simulink model "mpptwithANN"  (R2024b)
settings: Solver=VariableStepAuto  StartTime=0.0  StopTime=24.0  RelTol=1e-3
undefined symbols (not defined in the file): C_boost, f, L_boost, Lf, numericIrradiance, numericTemperature, PV_power_max, Ts, V_bus_ref
libraries: neural x84, slpidlib x3, spsSeriesRLCBranchLib x3, spsDiodeLib x1, spsIGBTLib x1, spsPLL3phLib x1, spsPWMGenerator2LevelLib x1, spsPower3phInstantaneousLib x1, spsTHDLib x1, spsabctodq0Lib x1, spsdq0toabcLib x1, spsThreePhaseSeriesRLCBranchLib x1
(part 3 of 3)

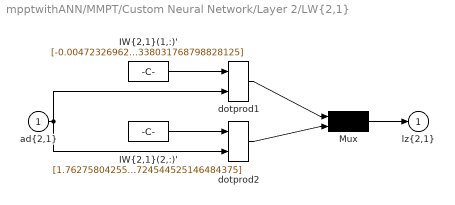
== system mpptwithANN/MMPT/Custom Neural Network/Layer 2/LW{2,1} ==
  "ad{2,1}" : Inport  PortDimensions=80
      mask Display: e = 0.06;c1 = [120 230 180]/255;c2 = ([120 230 180]+0)/(256+128);c3 = ([120 230 180]+128)/(256+128);patch([0 1 1 0],[0 0 1 1],c1);patch([0 1 1 1-e 1-e 0+e],[0 0 1 1-e 0+e 0+e],c2);patch([0 0 1 1-e 0+e 0+e],[0 1 1 1-e 1-e 0+e],c3);plot([0 1 1 0 0],[0 0 1 1 0]);
  "IW{2,1}(1,:)'" : Constant  Value=[-0.0047232696251935414599731899443213478662073612213134765625;-0.214237498205491594394089815978077240288257598876953125;-0.1861746145919385975187054782509221695363521575927734375;1.28709666919888210401268224813975393772125244140625;0.078470024721729980665685388885322026908397674560546875;1.731270590613536608515232728677801787853240966796875;1.00782466533039904987845147843472659587860107421875;1.6899709230974770957089958756114356219768524169921875;0.2274277742496670084992871352369547821581363677978515625;1.2774883926330662387016445791232399642467498779296875;1.2389200467032444041848293636576272547245025634765625;-0.6597367870607697692975079917232505977153778076171875;-0.06730057110412183962733223552277195267379283905029296875;0.24775995851258281188478349577053450047969818115234375;-1.264628121434770324782448369660414755344390869140625;0.11569644421095424957623976069953641854226589202880859375;-1.8753584133780234477484327726415358483791351318359375;0.71299671585435409060238498568651266396045684814453125;-0.6809653627305765066779486005543731153011322021484375;0.2444300914592904827582486859682830981910228729248046875;0.0794709997339119456061240498456754721701145172119140625;0.36944574372709626519650782938697375357151031494140625;0.88816890041603169247963478483143262565135955810546875;-0.02143380132873128063319967395727871917188167572021484375;0.50087358020141803383040723929298110306262969970703125;0.58260337805890072271353119504055939614772796630859375;-0.038040339388145251453554607223850325681269168853759765625;0.02344252262479391835103825769692775793373584747314453125;2.82094834954563111750758253037929534912109375;-0.04656330082969177552865147617922048084437847137451171875;1.098162614279721172039216980920173227787017822265625;0.462487932987993344280397423062822781503200531005859375;0.1327519260842389969834442808860330842435359954833984375;1.526963466155728088580190160428173840045928955078125;0.1184090589325994258285135174446622841060161590576171875;1.09930493106891535859404029906727373600006103515625;0.459243461526841978415092171417200006544589996337890625;0.040550115986065816964245556164314621128141880035400390625;0.0074893255565064709156075650753336958587169647216796875;-1.610216391686119852266756424796767532825469970703125;-0.260922289002195995077926227168063633143901824951171875;1.8914037685748421591114265538635663688182830810546875;0.029054511814582906215065349897486157715320587158203125;-1.291752843773599668253382333205081522464752197265625;-0.81151039446108785835320986734586767852306365966796875;-0.54747929068007616937308057458722032606601715087890625;0.6616069406555309395656649940065108239650726318359375;0.12428578364523527877150144149709376506507396697998046875;-0.0513260459514583156082068171599530614912509918212890625;0.26420608372235643290792950210743583738803863525390625;0.20916434229732139282731395724113099277019500732421875;-0.0612569342180534215369647199622704647481441497802734375;-1.011025237375536622863592128851450979709625244140625;0.2016605023533524221335255788289941847324371337890625;-0.070160014212906574027073247634689323604106903076171875;0.1338316497629020440651714807245298288762569427490234375;-0.1716200194942450185653370908767101354897022247314453125;-0.0084522613780383219761471735864688525907695293426513671875;-0.33277668814661753859951431877561844885349273681640625;0.40271319195953381164798656755010597407817840576171875;-1.693222936690923052793777969782240688800811767578125;2.97023091289202323395102212089113891124725341796875;0.60863251712745924937308927837875671684741973876953125;0.215351659861896804759595625000656582415103912353515625;0.199347225804359318157565894580329768359661102294921875;0.00390281946643264605889545038053256575949490070343017578125;0.155476210424553784594792205098201520740985870361328125;0.15170365314607192619433817526441998779773712158203125;0.07248701893488292136158435141624067910015583038330078125;1.544695222341591733794530227896757423877716064453125 ...(+582 chars)]
      mask Display: e = 0.06;c1 = [120 150 230]/255;c2 = ([120 150 230]+0)/383;c3 = ([120 150 230]+128)/383;patch([0 1 1 0],[0 0 1 1],c1);patch([0 1 1 1-e 1-e 0+e],[0 0 1 1-e 0+e 0+e],c2);patch([0 0 1 1-e 0+e 0+e],[0 1 1 1-e 1-e 0+e],c3);plot([0 1 1 0 0],[0 0 1 1 0]);disp('weights');
  "IW{2,1}(2,:)'" : Constant  Value=[1.7627580425513749151633646761183626949787139892578125;0.53943205208589140031705255751148797571659088134765625;0.624002903812199694044693387695588171482086181640625;-0.243051189123102251432584353096899576485157012939453125;1.1020632737466886652555331238545477390289306640625;-1.11695945169389698747863803873769938945770263671875;-0.98308582001807309769247922304202802479267120361328125;-0.057565707001347922455725125701064825989305973052978515625;1.0363818644077980035689279247890226542949676513671875;0.384261316616549664093582805435289628803730010986328125;0.3909105472417533366780162396025843918323516845703125;-1.7467929934915356060542990235262550413608551025390625;0.56609445637508437609852762761875055730342864990234375;0.265017689055616234572454459339496679604053497314453125;1.2954045387665560351564408847480081021785736083984375;-1.540932836613462253438910920522175729274749755859375;1.841363864427123520073337203939445316791534423828125;-0.305536607589804276585709885694086551666259765625;-1.13861542101164392448708895244635641574859619140625;1.625627574860612600815557016176171600818634033203125;2.8671914143540409014576653135009109973907470703125;0.346381542809648890202112170300097204744815826416015625;1.1745140811006609116162735517718829214572906494140625;-5.6920796134959150691656759590841829776763916015625;0.3262136683259966307701915866346098482608795166015625;-0.650348270424956353963352739810943603515625;3.41910464775504596701694026705808937549591064453125;-0.44059910956027170669813131098635494709014892578125;0.09728772033335808533394128971849568188190460205078125;2.2946392991425330620813838322646915912628173828125;-0.1401781681152533820533534481000970117747783660888671875;-6.91661892860060145693523736554197967052459716796875;1.0106115736624785572672635680646635591983795166015625;0.403771461315584889728569351063924841582775115966796875;1.5538543488356169053332678231527097523212432861328125;1.42685164398312824829417877481319010257720947265625;-0.669288812796880794309117845841683447360992431640625;0.64350597345122662051863926535588689148426055908203125;0.83719787664124101222995477655786089599132537841796875;0.504352515289591796232571141445077955722808837890625;-1.3964692966659886241842514209565706551074981689453125;-2.366240715256571203184421392506919801235198974609375;1.3210995760871833137883868403150700032711029052734375;-1.6112503545807108640275373545591719448566436767578125;-0.61634350787260683279811246393364854156970977783203125;-0.67204202473365326486742787892580963671207427978515625;-1.3503900477962533788200971685000695288181304931640625;1.8406531941525015039218260426423512399196624755859375;-0.55840708318073328797481735819019377231597900390625;-1.3308330118435793831821456478792242705821990966796875;1.08996733967639869433696730993688106536865234375;-1.2525754013379206686096267731045372784137725830078125;1.015163588563302798917220570729114115238189697265625;-0.494342640937765087638666727798408828675746917724609375;1.3083195368033699867993391308118589222431182861328125;-1.6629750494247514946977162253460846841335296630859375;-0.64384781628943965614553235354833304882049560546875;0.2008878295447505124560194644800503738224506378173828125;0.9673933358097617229987008613534271717071533203125;-0.30449682571478497994377221402828581631183624267578125;0.8817019505081702401838583682547323405742645263671875;1.688775129151605103317024259013123810291290283203125;-0.35288033498891213657344678722438402473926544189453125;-0.64764787986383531848133543462608940899372100830078125;-2.5027077798869736824372012051753699779510498046875;1.4127423164830534840774589611100964248180389404296875;-0.870574382676529534563769630040042102336883544921875;-0.58183267759664081264503465718007646501064300537109375;-1.5020935863691480260939670188236050307750701904296875;0.74543326788178509989535314161912538111209869384765625;0.218338872138691131308263493338017724454402923583984375;-0.951693733442773304176398596609942615032196044921875 ...(+447 chars)]
      mask Display: e = 0.06;c1 = [120 150 230]/255;c2 = ([120 150 230]+0)/383;c3 = ([120 150 230]+128)/383;patch([0 1 1 0],[0 0 1 1],c1);patch([0 1 1 1-e 1-e 0+e],[0 0 1 1-e 0+e 0+e],c2);patch([0 0 1 1-e 0+e 0+e],[0 1 1 1-e 1-e 0+e],c3);plot([0 1 1 0 0],[0 0 1 1 0]);disp('weights');
  Mux : Mux  Inputs=2
      mask Display: e = 0.06;c1 = [120 150 230]/255;c2 = ([120 150 230]+0)/383;c3 = ([120 150 230]+128)/383;patch([0 1 1 0],[0 0 1 1],c1);patch([0 1 1 1-e 1-e 0+e],[0 0 1 1-e 0+e 0+e],c2);patch([0 0 1 1-e 0+e 0+e],[0 1 1 1-e 1-e 0+e],c3);plot([0 1 1 0 0],[0 0 1 1 0]);disp('Mux');
  dotprod1 : neural/Weight Functions/dotprod
  dotprod2 : neural/Weight Functions/dotprod
  "lz{2,1}" : Outport
      mask Display: e = 0.06;c1 = [120 230 180]/255;c2 = ([120 230 180]+0)/(256+128);c3 = ([120 230 180]+128)/(256+128);patch([0 1 1 0],[0 0 1 1],c1);patch([0 1 1 1-e 1-e 0+e],[0 0 1 1-e 0+e 0+e],c2);patch([0 0 1 1-e 0+e 0+e],[0 1 1 1-e 1-e 0+e],c3);plot([0 1 1 0 0],[0 0 1 1 0]);
  wires:
  "IW{2,1}(1,:)'"/1 -> dotprod1/1
  "ad{2,1}"/1 -> dotprod1/2, dotprod2/2
  dotprod1/1 -> Mux/1
  "IW{2,1}(2,:)'"/1 -> dotprod2/1
  dotprod2/1 -> Mux/2
  Mux/1 -> "lz{2,1}"/1

== matlab function mpptwithANN/MMPT/MATLAB Function ==
  data: I input; V input; inputs output
function inputs = processSignals(I, V)
%#codegen

% Inputs:
% I: Structure containing Time and Data for current
% V: Structure containing Time and Data for voltage

% Outputs:
% inputs: Matrix with [time, V_data, I_data] after downsampling

    % Extract time and data
    I_time = I.Time;       % Time for current
    I_data = I.Data;       % Current values

    V_time = V.Time;       % Time for voltage
    V_data = V.Data;       % Voltage values

    % Downsample the data
    downsampleRate = 1000;
    Idata = I_data(1:downsampleRate:end);
    Vdata = V_data(1:downsampleRate:end);
    time = V_time(1:downsampleRate:end);

    % Prepare input vector
    inputs = [time, Vdata, Idata]'; % Input matrix
end
